simulink model "VCMGCM1962020b_v2"  (R2020b)
settings: Solver=FixedStepDiscrete  StartTime=0.0  StopTime=10.0  FixedStep=0.005  RelTol=1e-3  EnableMultiTasking=on
PreLoadFcn:
  | try, model_open; catch, disp('Error occurred while executing model pre-load callback: model_open.m'); disp('Please assure that the MATLAB working directory is set to the model directory before opening.'); end
InitFcn:
  | try, model_open; catch, end
undefined symbols (not defined in the file): Bridge, GCM, H, raptor_get_param_eval, raptor_get_safe_string, raptor_xcp_function
libraries: Blocks_lib x1165, Raptor_lib x665, simulink x62, VCM_lib x5
(part 9 of 23)

== system VCMGCM1962020b_v2/Fgnd/Control/PDU/Main  Contactor Cmd/HV Detect ==
  Data : Inport
  Abs : Abs
  Add : Sum  Inputs=+-  InputSameDT=on  OutDataTypeStr=Inherit: Same as first input
  Bus Selector : BusSelector  OutputSignals=VirtualSensors.PDU.HVBusVolt [V]
  Bus Selector1 : BusSelector  OutputSignals=VirtualSensors.Batt.BattVolt [V]
  Header : Blocks_lib/Header  width=Portrait  addtext=''
  Logical Operator : Logic  AllPortsSameDT=off  OutDataTypeStr=boolean
  Relational Operator : RelationalOperator  OutDataTypeStr=boolean  RndMeth=Nearest
  Relational Operator1 : RelationalOperator  Operator=<=  OutDataTypeStr=boolean  RndMeth=Nearest
  raptor_adjustment : Raptor_lib/Data Storage/raptor_adjustment  paramName=[nam 'PreChgHVDetectThr']  nameSource=Parameter  initValue=0  dataType=double  storage=Calibration  calDispType=Number  calEnum={'Disabled', 'Enabled'}  calGain=1  calOffset=0  calMax=inf  calMin=-inf  calFormat=''  calUnit='V'  calHelp='Pre-charge high voltage detected threshold (post contactors)'  calAccess=1  calFunction=group  calDispHeaders=off  calColHeaders={'Col1' 'Col2' 'Col3'}  calRowHeaders={'Row1' 'Row2' 'Row3'}
      settings: SourceProductName=Raptor
  raptor_adjustment1 : Raptor_lib/Data Storage/raptor_adjustment  paramName=[nam 'PreChgHVDetectDeltaThr']  nameSource=Parameter  initValue=0  dataType=double  storage=Calibration  calDispType=Number  calEnum={'Disabled', 'Enabled'}  calGain=1  calOffset=0  calMax=inf  calMin=-inf  calFormat=''  calUnit='V'  calHelp='Pre-charge high voltage detected threshold (delta between pre and post contactors)'  calAccess=1  calFunction=group  calDispHeaders=off  calColHeaders={'Col1' 'Col2' 'Col3'}  calRowHeaders={'Row1' 'Row2' 'Row3'}
      settings: SourceProductName=Raptor
  raptor_measurement : Raptor_lib/Data Storage/raptor_measurement  paramName=[nam 'HVDetect']  nameSource=Parameter  calDispType=Number  calEnum={'Disabled', 'Enabled'}  calGain=1  calOffset=0  calMax=inf  calMin=-inf  calFormat=''  calUnit='Bool'  calHelp='high voltage detected (post contactors)'  calAccess=1  calFunction=group  calVisible=on
      settings: SourceProductName=Raptor
  Full : Outport  VectorParamsAs1DForOutWhenUnconnected=off
  wires:
  raptor_adjustment1/1 -> Relational Operator1/2
  Relational Operator1/1 -> Logical Operator/2
  Relational Operator/1 -> Logical Operator/1
  Add/1 -> Abs/1
  raptor_adjustment/1 -> Relational Operator/2
  Bus Selector1/1 -> Add/2  "<BattVolt [V]>"
  Abs/1 -> Relational Operator1/1
  Logical Operator/1 -> Full/1, raptor_measurement/1
  Data/1 -> Bus Selector1/1, Bus Selector/1
  Bus Selector/1 -> Relational Operator/1, Add/1  "<HVBusVolt [V]>"

== system VCMGCM1962020b_v2/Fgnd/Control/PDU/Main  Contactor Cmd/PreCharge Sequence/EvalDiag ==
  status : Inport
  f : TriggerPort  TriggerType=function-call  VariantControl=(inherit)
      settings: CopyFcn=Stateflow.SLINSF.SimulinkMan.removeBlockPreDeleteFcn  PreDeleteFcn=Stateflow.SLINSF.SimulinkMan.unsafePredeleteFcn
  Header : Blocks_lib/Header  width=Portrait  addtext=''
  raptor_fault_def : Raptor_lib/Faults/raptor_fault_def  faultName=[nam 'PreChgFault']  persist=off  sticky=off  emisRelated=off  singleTrip=off  clearMethod=Standard  xLimit=1  yLimit=1  calEnable=on  addDisable=off  calAccess=1  calFunction=['Diagnostics | Fault Defs | ' raptor_get_param_eval(gcb, 'faultName')]
      settings: SourceProductName=Raptor
  wires:
  status/1 -> raptor_fault_def/1

== system VCMGCM1962020b_v2/Fgnd/Control/PDU/PDU Contactor Commands/CntrStatus ==
  Data : Inport
  AND : Logic  Inputs=4  AllPortsSameDT=off  OutDataTypeStr=boolean
  AND1 : Logic  Inputs=4  AllPortsSameDT=off  OutDataTypeStr=boolean
  Bus Selector : BusSelector  OutputSignals=Sensors.Sensors.Other.DrvInvtrCntrClosed.DrvInvtrCntrClosed [Bool],Sensors.Sensors.Other.DCDCCntrClosed.DCDCCntrClosedVld [Bool],Sensors.Sensors.Other.DCDCCntrClosed.DCDCCntrClosed [Bool],Sensors.Sensors.Other.ChrgrCntrClosed.ChrgrCntrClosedVld [Bool]
  Bus Selector1 : BusSelector  OutputSignals=Sensors.Sensors.Other.ChrgrCntrClosed.ChrgrCntrClosedVld [Bool],Sensors.Sensors.Other.ChrgrCntrClosed.ChrgrCntrClosed [Bool]
  Header : Blocks_lib/Header  width=Portrait  addtext=''
  Meas&Ovrd1 : Blocks_lib/Meas&Ovrd  nam='RunCntrClosed'  name_source=Parameter  view_as=Number  enum_struct={}  gain=1  min=-inf  max=inf  precision=''  units='Bool'  help='Run Contactor state'  group='Control | PDU'
  Meas&Ovrd10 : Blocks_lib/Meas&Ovrd  nam='ChrgCntrClosed'  name_source=Parameter  view_as=Number  enum_struct={}  gain=1  min=-inf  max=inf  precision=''  units='Bool'  help='Charge Contactor state'  group='Control | PDU'
  RunClosed : Outport  VectorParamsAs1DForOutWhenUnconnected=off
  ChrgClosed : Outport  Port=2  VectorParamsAs1DForOutWhenUnconnected=off
  wires:
  Data/1 -> Bus Selector1/1, Bus Selector/1
  AND1/1 -> Meas&Ovrd10/1
  AND/1 -> Meas&Ovrd1/1
  Bus Selector/1 -> AND/1  "<DrvInvtrCntrClosed [Bool]>"
  Bus Selector/2 -> AND/2  "<DCDCCntrClosedVld [Bool]>"
  Bus Selector/3 -> AND1/1, AND/3  "<DCDCCntrClosed [Bool]>"
  Bus Selector/4 -> AND1/2, AND/4  "<ChrgrCntrClosedVld [Bool]>"
  Bus Selector1/1 -> AND1/3  "<ChrgrCntrClosedVld [Bool]>"
  Bus Selector1/2 -> AND1/4  "<ChrgrCntrClosed [Bool]>"
  Meas&Ovrd10/1 -> ChrgClosed/1
  Meas&Ovrd1/1 -> RunClosed/1

== system VCMGCM1962020b_v2/Fgnd/Control/PDU/PDU Contactor Commands/Drive Inverter Contactor ==
  Data : Inport
  Abs : Abs
  Bus Selector : BusSelector  OutputSignals=Control.Mode.StartStop.RunCntr [Bool]
  Bus Selector1 : BusSelector  OutputSignals=VirtualSensors.DrvInvtr.DrvMtrSpd [rpm]
  Header : Blocks_lib/Header  width=Portrait  addtext=''
  Logical Operator : Logic  Operator=OR  AllPortsSameDT=off  OutDataTypeStr=boolean
  Logical Operator1 : Logic  Operator=NOT  Inputs=1  AllPortsSameDT=off  OutDataTypeStr=boolean
  Logical Operator2 : Logic  OutDataTypeStr=boolean
  Meas&Ovrd10 : Blocks_lib/Meas&Ovrd  nam='DrvCntrCmd'  name_source=Parameter  view_as=Number  enum_struct={}  gain=1  min=-inf  max=inf  precision=''  units='Bool'  help='Drive Contactor state'  group='Control | PDU'
  Relational Operator : RelationalOperator  Operator=>  OutDataTypeStr=boolean  RndMeth=Simplest
  Set : Blocks_lib/Set  SystemSampleTime=-1  VariantActivationTime=update diagram  Latency=0  AutoFrameSizeCalculation=off
  raptor_adjustment : Raptor_lib/Data Storage/raptor_adjustment  paramName='DrvInvtrCntrDsblMtrSpdThr'  nameSource=Parameter  initValue=0  dataType=double  storage=Calibration  calDispType=Number  calEnum={'False', 'True'}  calGain=1.0  calOffset=0.0  calMax=inf  calMin=-inf  calFormat=''  calUnit='rpm'  calHelp='Drive inverter contactor disable threshold (on motor speed, during HV discharge)'  calAccess=1  calFunction='Control | PDU'  calDispHeaders=off  calColHeaders={'Col1' 'Col2' 'Col3'}  calRowHeaders={'Row1' 'Row2' 'Row3'}
      settings: SourceProductName=Raptor
  raptor_fault_status : Raptor_lib/Faults/raptor_fault_status  faultSource=Parameter  faultName='EStop1'  notOccurred=off  suspected=off  active=off  occurred=off  failedThisDC=on  testCmpltThisDC=off  failing=off  pending=off  confirmed=off  mil=off  permanent=off  ready=off  prevConfirmed=off  failedSinceClear=off  failedLastDC=off  prevMil=off
      settings: SourceProductName=Raptor
  Bool : Outport  VectorParamsAs1DForOutWhenUnconnected=off
  wires:
  raptor_adjustment/1 -> Relational Operator/2
  Bus Selector1/1 -> Abs/1  "<DrvMtrSpd [rpm]>"
  Data/1 -> Bus Selector1/1, Bus Selector/1
  Abs/1 -> Relational Operator/1
  Bus Selector/1 -> Logical Operator2/1  "<RunCntr [Bool]>"
  Meas&Ovrd10/1 -> Bool/1
  Logical Operator2/1 -> Meas&Ovrd10/1
  Relational Operator/1 -> Logical Operator/1
  raptor_fault_status/1 -> Logical Operator/2
  Logical Operator/1 -> Set/1
  Set/1 -> Logical Operator1/1
  Logical Operator1/1 -> Logical Operator2/2

== system VCMGCM1962020b_v2/Fgnd/Control/PDU/PDU Contactor Commands/Enable ==
  Data : Inport
  Bus Selector : BusSelector  OutputSignals=Control.Mode.StartStop.RunCntr [Bool],Control.Mode.StartStop.ChgCntr [Bool]
  Header : Blocks_lib/Header  width=Portrait  addtext=''
  Logical Operator : Logic  Operator=NOT  Inputs=1  AllPortsSameDT=off  OutDataTypeStr=boolean
  Logical Operator1 : Logic  AllPortsSameDT=off  OutDataTypeStr=boolean
  Logical Operator2 : Logic  AllPortsSameDT=off  OutDataTypeStr=boolean
  raptor_fault_status : Raptor_lib/Faults/raptor_fault_status  faultSource=Parameter  faultName='EStop1'  notOccurred=off  suspected=off  active=off  occurred=off  failedThisDC=on  testCmpltThisDC=off  failing=off  pending=off  confirmed=off  mil=off  permanent=off  ready=off  prevConfirmed=off  failedSinceClear=off  failedLastDC=off  prevMil=off
      settings: SourceProductName=Raptor
  RunEnbl : Outport  VectorParamsAs1DForOutWhenUnconnected=off
  ChrgEnbl : Outport  Port=2  VectorParamsAs1DForOutWhenUnconnected=off
  wires:
  Logical Operator1/1 -> RunEnbl/1
  Data/1 -> Bus Selector/1
  Logical Operator/1 -> Logical Operator2/1, Logical Operator1/1
  raptor_fault_status/1 -> Logical Operator/1
  Bus Selector/1 -> Logical Operator1/2  "<RunCntr [Bool]>"
  Bus Selector/2 -> Logical Operator2/2  "<ChgCntr [Bool]>"
  Logical Operator2/1 -> ChrgEnbl/1

== system VCMGCM1962020b_v2/Fgnd/Control/PDU/PDU Contactor Commands/HV Detect ==
  Data : Inport
  Abs : Abs
  Add : Sum  Inputs=+-  InputSameDT=on  OutDataTypeStr=Inherit: Same as first input
  Bus Selector : BusSelector  OutputSignals=VirtualSensors.PDU.HVBusVolt [V]
  Bus Selector1 : BusSelector  OutputSignals=VirtualSensors.Batt.BattVolt [V]
  Header : Blocks_lib/Header  width=Portrait  addtext=''
  Logical Operator : Logic  AllPortsSameDT=off  OutDataTypeStr=boolean
  Relational Operator : RelationalOperator  OutDataTypeStr=boolean  RndMeth=Nearest
  Relational Operator1 : RelationalOperator  Operator=<=  OutDataTypeStr=boolean  RndMeth=Nearest
  raptor_adjustment : Raptor_lib/Data Storage/raptor_adjustment  paramName=['PreChgHVDetectThr']  nameSource=Parameter  initValue=0  dataType=double  storage=Calibration  calDispType=Number  calEnum={'Disabled', 'Enabled'}  calGain=1  calOffset=0  calMax=inf  calMin=-inf  calFormat=''  calUnit='V'  calHelp='Pre-charge high voltage detected threshold (post contactors)'  calAccess=1  calFunction=group  calDispHeaders=off  calColHeaders={'Col1' 'Col2' 'Col3'}  calRowHeaders={'Row1' 'Row2' 'Row3'}
      settings: SourceProductName=Raptor
  raptor_adjustment1 : Raptor_lib/Data Storage/raptor_adjustment  paramName=['PreChgHVDetectDeltaThr']  nameSource=Parameter  initValue=0  dataType=double  storage=Calibration  calDispType=Number  calEnum={'Disabled', 'Enabled'}  calGain=1  calOffset=0  calMax=inf  calMin=-inf  calFormat=''  calUnit='V'  calHelp='Pre-charge high voltage detected threshold (delta between pre and post contactors)'  calAccess=1  calFunction=group  calDispHeaders=off  calColHeaders={'Col1' 'Col2' 'Col3'}  calRowHeaders={'Row1' 'Row2' 'Row3'}
      settings: SourceProductName=Raptor
  raptor_measurement : Raptor_lib/Data Storage/raptor_measurement  paramName=['HVDetect']  nameSource=Parameter  calDispType=Number  calEnum={'Disabled', 'Enabled'}  calGain=1  calOffset=0  calMax=inf  calMin=-inf  calFormat=''  calUnit='Bool'  calHelp='high voltage detected (post contactors)'  calAccess=1  calFunction=group  calVisible=on
      settings: SourceProductName=Raptor
  Full : Outport  VectorParamsAs1DForOutWhenUnconnected=off
  wires:
  raptor_adjustment1/1 -> Relational Operator1/2
  Relational Operator1/1 -> Logical Operator/2
  Relational Operator/1 -> Logical Operator/1
  Add/1 -> Abs/1
  raptor_adjustment/1 -> Relational Operator/2
  Bus Selector1/1 -> Add/2  "<BattVolt [V]>"
  Abs/1 -> Relational Operator1/1
  Logical Operator/1 -> Full/1, raptor_measurement/1
  Data/1 -> Bus Selector1/1, Bus Selector/1
  Bus Selector/1 -> Relational Operator/1, Add/1  "<HVBusVolt [V]>"

== system VCMGCM1962020b_v2/Fgnd/Diagnostics/Diagnostics/A//C Compressor Fault/EvalDiag ==
  note: Note: under-voltage or internal fault are only considered a fault
      | when contactors are closed.
  Data : Inport
  Reset : EnablePort  StatesWhenEnabling=reset
  Bus Selector : BusSelector  OutputSignals=Sensors.CAN.Other.ACC.ACCSTATUS1.ACCFltStat.ACCFltStat []
  Bus Selector1 : BusSelector  OutputSignals=VirtualSensors.PDU.MainCntrClosed [Bool]
  FltTmr : Blocks_lib/FltTmr  nam='ACCFault'  tmrth_nam='ACCFaultTimeThr'  tmrth_typ=uint16  tmrth_help='Fault time threshold'  samptime=samptime  group='Diagnostics | System'
  Header : Blocks_lib/Header  width=Portrait  addtext=''
  Internal Fault : simulink/Logic and Bit Operations/Compare To Constant  relop===  const=6  OutDataTypeStr=boolean
  Logical Operator : Logic  AllPortsSameDT=off  OutDataTypeStr=boolean
  Logical Operator1 : Logic  Operator=OR  AllPortsSameDT=off  OutDataTypeStr=boolean
  Logical Operator2 : Logic  AllPortsSameDT=off  OutDataTypeStr=boolean
  Logical Operator3 : Logic  Operator=OR  AllPortsSameDT=off  OutDataTypeStr=boolean
  Logical Operator4 : Logic  Operator=NOT  AllPortsSameDT=off  OutDataTypeStr=boolean
  No Fault : simulink/Logic and Bit Operations/Compare To Zero  relop=~=  OutDataTypeStr=boolean
  Under Voltage : simulink/Logic and Bit Operations/Compare To Constant  relop===  const=1  OutDataTypeStr=boolean
  wires:
  Data/1 -> Bus Selector/1, Bus Selector1/1
  Internal Fault/1 -> Logical Operator3/2
  No Fault/1 -> Logical Operator/1
  Logical Operator/1 -> Logical Operator1/1
  Logical Operator2/1 -> Logical Operator1/2
  Under Voltage/1 -> Logical Operator3/1
  Logical Operator3/1 -> Logical Operator2/1, Logical Operator4/1
  Bus Selector1/1 -> Logical Operator2/2  "<MainCntrClosed [Bool]>"
  Logical Operator4/1 -> Logical Operator/2
  Logical Operator1/1 -> FltTmr/1
  Bus Selector/1 -> Internal Fault/1, Under Voltage/1, No Fault/1  "<ACCFltStat []>"

== system VCMGCM1962020b_v2/Fgnd/Diagnostics/Diagnostics/Battery Cell Temperature (avg) High /EvalDiag ==
  Data : Inport
  Reset : EnablePort  StatesWhenEnabling=reset
  Bus Selector : BusSelector  OutputSignals=VirtualSensors.Batt.BattCellTempAvg [degC]
  FltRngTmr : Blocks_lib/FltRngTmr  nam='BattCellTempAvgHi'  relop=>  threshnam='BattCellTempAvgHiThr'  typ=double  units='degC'  help='Range high fault threshold'  tmrth_nam='BattCellTempAvgHiTimeThr'  tmrth_typ=uint16  tmrth_help='Range high fault time threshold'  samptime=samptime  group='Diagnostics | System'
  Header : Blocks_lib/Header  width=Portrait  addtext=''
  wires:
  Data/1 -> Bus Selector/1
  Bus Selector/1 -> FltRngTmr/1  "<BattCellTempAvg [degC]>"

== system VCMGCM1962020b_v2/Fgnd/Diagnostics/Diagnostics/Battery Cell Temperature (max) High/EvalDiag ==
  Data : Inport
  Reset : EnablePort  StatesWhenEnabling=reset
  Bus Selector : BusSelector  OutputSignals=VirtualSensors.Batt.BattCellTempMx [degC]
  FltRngTmr : Blocks_lib/FltRngTmr  nam='BattCellTempMxHi'  relop=>  threshnam='BattCellTempMxHiThr'  typ=double  units='degC'  help='Range high fault threshold'  tmrth_nam='BattCellTempMxHiTimeThr'  tmrth_typ=uint16  tmrth_help='Range high fault time threshold'  samptime=samptime  group='Diagnostics | System'
  Header : Blocks_lib/Header  width=Portrait  addtext=''
  wires:
  Bus Selector/1 -> FltRngTmr/1  "<BattCellTempMx [degC]>"
  Data/1 -> Bus Selector/1

== system VCMGCM1962020b_v2/Fgnd/Diagnostics/Diagnostics/Battery Cell Voltage (max) High/EvalDiag ==
  Data : Inport
  Reset : EnablePort  StatesWhenEnabling=reset
  Bus Selector : BusSelector  OutputSignals=VirtualSensors.Batt.BattCellVoltMx [V]
  FltRngTmr : Blocks_lib/FltRngTmr  nam='BattCellVoltMxHi'  relop=>  threshnam='BattCellVoltMxHiThr'  typ=double  units='V'  help='Range high fault threshold'  tmrth_nam='BattCellVoltMxHiTimeThr'  tmrth_typ=uint16  tmrth_help='Range high fault time threshold'  samptime=samptime  group='Diagnostics | System'
  Header : Blocks_lib/Header  width=Portrait  addtext=''
  wires:
  Bus Selector/1 -> FltRngTmr/1  "<BattCellVoltMx [V]>"
  Data/1 -> Bus Selector/1

== system VCMGCM1962020b_v2/Fgnd/Diagnostics/Diagnostics/Battery Cell Voltage (min) Low/EvalDiag ==
  Data : Inport
  Reset : EnablePort  StatesWhenEnabling=reset
  Bus Selector : BusSelector  OutputSignals=VirtualSensors.Batt.BattCellVoltMn [V]
  FltRngTmr : Blocks_lib/FltRngTmr  nam='BattCellVoltMnLo'  relop=<  threshnam='BattCellVoltMnLoThr'  typ=double  units='V'  help='Range low fault threshold'  tmrth_nam='BattCellVoltMnLoTimeThr'  tmrth_typ=uint16  tmrth_help='Range low fault time threshold'  samptime=samptime  group='Diagnostics | System'
  Header : Blocks_lib/Header  width=Portrait  addtext=''
  wires:
  Data/1 -> Bus Selector/1
  Bus Selector/1 -> FltRngTmr/1  "<BattCellVoltMn [V]>"

== system VCMGCM1962020b_v2/Fgnd/Diagnostics/Diagnostics/Battery Current High/EvalDiag ==
  Data : Inport
  Reset : EnablePort  StatesWhenEnabling=reset
  Add : Sum
  Add1 : Sum
  Bus Selector1 : BusSelector  OutputSignals=VirtualSensors.Batt.BattCur [A]
  Bus Selector2 : BusSelector  OutputSignals=VirtualSensors.Batt.BattCCL [A]
  Bus Selector9 : BusSelector  OutputSignals=VirtualSensors.Batt.BattDCL [A]
  FltTmr : Blocks_lib/FltTmr  nam='BattCurHi'  tmrth_nam='BattCurHiTimeThr'  tmrth_typ=uint16  tmrth_help='Range high fault time threshold'  samptime=samptime  group='Diagnostics | System'
  Gain : Gain  Gain=-1
  Header : Blocks_lib/Header  width=Portrait  addtext=''
  Logical Operator : Logic  Operator=OR  OutDataTypeStr=boolean
  Relational Operator : RelationalOperator  Operator=>  OutDataTypeStr=boolean  RndMeth=Nearest  InputSameDT=on
  Relational Operator1 : RelationalOperator  Operator=<  OutDataTypeStr=boolean  RndMeth=Nearest  InputSameDT=on
  raptor_adjustment1 : Raptor_lib/Data Storage/raptor_adjustment  paramName='BattCurHiThrHyst'  nameSource=Parameter  initValue=0  dataType=double  storage=Calibration  calDispType=Number  calEnum={'Disabled', 'Enabled'}  calGain=1  calOffset=0  calMax=inf  calMin=-inf  calFormat=''  calUnit='A'  calHelp='Range high fault threshold hysteresis (on limits)'  calAccess=1  calFunction='Diagnostics | System'  calDispHeaders=off  calColHeaders={'Col1' 'Col2' 'Col3'}  calRowHeaders={'Row1' 'Row2' 'Row3'}
      settings: SourceProductName=Raptor
  wires:
  Add1/1 -> Gain/1
  Relational Operator/1 -> Logical Operator/1
  Relational Operator1/1 -> Logical Operator/2
  Bus Selector1/1 -> Relational Operator1/1, Relational Operator/1  "<BattCur [A]>"
  Add/1 -> Relational Operator/2
  raptor_adjustment1/1 -> Add1/2, Add/2
  Bus Selector9/1 -> Add/1  "<BattDCL [A]>"
  Bus Selector2/1 -> Add1/1  "<BattCCL [A]>"
  Logical Operator/1 -> FltTmr/1
  Gain/1 -> Relational Operator1/2
  Data/1 -> Bus Selector9/1, Bus Selector2/1, Bus Selector1/1

== system VCMGCM1962020b_v2/Fgnd/Diagnostics/Diagnostics/Battery Fault/EvalDiag ==
  Data : Inport
  Reset : EnablePort  StatesWhenEnabling=reset
  Bus Selector : BusSelector  OutputSignals=VirtualSensors.Batt.BattFault [Bool]
  FltTmr : Blocks_lib/FltTmr  nam='BattFault'  tmrth_nam='BattFaultTimeThr'  tmrth_typ=uint16  tmrth_help='Fault time threshold'  samptime=samptime  group='Diagnostics | System'
  Header : Blocks_lib/Header  width=Portrait  addtext=''
  wires:
  Data/1 -> Bus Selector/1
  Bus Selector/1 -> FltTmr/1  "<BattFault [Bool]>"

== system VCMGCM1962020b_v2/Fgnd/Diagnostics/Diagnostics/CAN Bus Passive/EvalDiag ==
  Reset : EnablePort  StatesWhenEnabling=reset
  CAN1 : Subsystem  mask{bus='CAN1'}
      mask prompts: bus "CAN Bus"
      mask init:
      | cb = gcb;
      | 
      | % --- Parameter Setting
      | set_param([cb '/raptor_can_state'], 'resource', bus);
      | set_param([cb '/raptor_can_tx_queue_info'], 'resource', bus);
      | set_param([cb '/raptor_can_tx_queue_info1'], 'resource', bus);
      mask Display: disp(bus)
  CAN2 : Subsystem  Commented=on  mask{bus='CAN2'}
      mask prompts: bus "CAN Bus"
      mask init: same as VCMGCM1962020b_v2/Fgnd/Diagnostics/Diagnostics/CAN Bus Passive/EvalDiag/CAN1
      mask Display: disp(bus)
  CAN3 : Subsystem  mask{bus='CAN3'}
      mask prompts: bus "CAN Bus"
      mask init: same as VCMGCM1962020b_v2/Fgnd/Diagnostics/Diagnostics/CAN Bus Passive/EvalDiag/CAN1
      mask Display: disp(bus)
  Header : Blocks_lib/Header  width=Portrait  addtext=''

== system VCMGCM1962020b_v2/Fgnd/Diagnostics/Diagnostics/Charger (off-board) Isolation Fault/EvalDiag ==
  Data : Inport
  Reset : EnablePort  StatesWhenEnabling=reset
  Bus Selector : BusSelector  OutputSignals=VirtualSensors.Chgr.OffBoard.OffBoardChgrIsoFault [Bool]
  FltTmr : Blocks_lib/FltTmr  nam='OffBoardChgrIsoFault'  tmrth_nam='OffBoardChgrIsoFaultTimeThr'  tmrth_typ=uint16  tmrth_help='Fault time threshold'  samptime=samptime  group='Diagnostics | System'
  Header : Blocks_lib/Header  width=Portrait  addtext=''
  wires:
  Bus Selector/1 -> FltTmr/1  "<OffBoardChgrIsoFault [Bool]>"
  Data/1 -> Bus Selector/1

== system VCMGCM1962020b_v2/Fgnd/Diagnostics/Diagnostics/Charger (on-board) Fault/EvalDiag ==
  Data : Inport
  Reset : EnablePort  StatesWhenEnabling=reset
  Bus Selector : BusSelector  OutputSignals=VirtualSensors.Chgr.OnBoard.OnBoardChgrFault [Bool]
  FltTmr : Blocks_lib/FltTmr  nam='OnBoardChgrFault'  tmrth_nam='OnBoardChgrFaultTimeThr'  tmrth_typ=uint16  tmrth_help='Fault time threshold'  samptime=samptime  group='Diagnostics | System'
  Header : Blocks_lib/Header  width=Portrait  addtext=''
  wires:
  Bus Selector/1 -> FltTmr/1  "<OnBoardChgrFault [Bool]>"
  Data/1 -> Bus Selector/1

== system VCMGCM1962020b_v2/Fgnd/Diagnostics/Diagnostics/Contactor X-Checks/EvalDiagChgrCntr ==
  Data : Inport
  Reset : EnablePort  StatesWhenEnabling=reset
  Bus Selector : BusSelector  OutputSignals=Control.PDU.PDUCntrs.ChrgrCntrCmd [Bool],VirtualSensors.PDU.ChrgrCntrClosed [Bool]
  FltTmr : Blocks_lib/FltTmr  nam='DCChgNegCntrXChk'  tmrth_nam='DCChgNegCntrXChkTimeThr'  tmrth_typ=uint16  tmrth_help='Cross-check fault time threshold'  samptime=samptime  group='Diagnostics | System'
  Header : Blocks_lib/Header  width=Portrait  addtext=''
  Logical Operator : Logic  Operator=NOT  Inputs=1  OutDataTypeStr=boolean
  Logical Operator1 : Logic  Operator=NOT  Inputs=1  OutDataTypeStr=boolean
  Logical Operator2 : Logic  OutDataTypeStr=boolean
  Logical Operator3 : Logic  OutDataTypeStr=boolean
  Logical Operator4 : Logic  Operator=OR  OutDataTypeStr=boolean
  wires:
  Data/1 -> Bus Selector/1
  Logical Operator1/1 -> Logical Operator3/1
  Logical Operator3/1 -> Logical Operator4/2
  Logical Operator2/1 -> Logical Operator4/1
  Logical Operator/1 -> Logical Operator2/2
  Bus Selector/1 -> Logical Operator2/1, Logical Operator1/1  "<ChrgrCntrCmd [Bool]>"
  Bus Selector/2 -> Logical Operator3/2, Logical Operator/1  "<ChrgrCntrClosed [Bool]>"
  Logical Operator4/1 -> FltTmr/1

== system VCMGCM1962020b_v2/Fgnd/Diagnostics/Diagnostics/Contactor X-Checks/EvalDiagDCDCCntr ==
  Data : Inport
  Reset : EnablePort  StatesWhenEnabling=reset
  Bus Selector : BusSelector  OutputSignals=VirtualSensors.PDU.DCDCCntrClosed [Bool],Control.PDU.PDUCntrs.DCDCCntrCmd [Bool]
  FltTmr : Blocks_lib/FltTmr  nam='DCChgPosCntrXChk'  tmrth_nam='DCChgPosCntrXChkTimeThr'  tmrth_typ=uint16  tmrth_help='Cross-check fault time threshold'  samptime=samptime  group='Diagnostics | System'
  Header : Blocks_lib/Header  width=Portrait  addtext=''
  Logical Operator : Logic  Operator=NOT  Inputs=1  OutDataTypeStr=boolean
  Logical Operator1 : Logic  Operator=NOT  Inputs=1  OutDataTypeStr=boolean
  Logical Operator2 : Logic  OutDataTypeStr=boolean
  Logical Operator3 : Logic  OutDataTypeStr=boolean
  Logical Operator4 : Logic  Operator=OR  OutDataTypeStr=boolean
  wires:
  Logical Operator4/1 -> FltTmr/1
  Bus Selector/2 -> Logical Operator/1, Logical Operator3/2  "<DCDCCntrCmd [Bool]>"
  Bus Selector/1 -> Logical Operator1/1, Logical Operator2/1  "<DCDCCntrClosed [Bool]>"
  Logical Operator/1 -> Logical Operator2/2
  Logical Operator2/1 -> Logical Operator4/1
  Logical Operator3/1 -> Logical Operator4/2
  Logical Operator1/1 -> Logical Operator3/1
  Data/1 -> Bus Selector/1

== system VCMGCM1962020b_v2/Fgnd/Diagnostics/Diagnostics/Contactor X-Checks/EvalDiagDrvInvtrCntr ==
  Data : Inport
  Reset : EnablePort  StatesWhenEnabling=reset
  Bus Selector : BusSelector  OutputSignals=VirtualSensors.PDU.DrvInvtrCntrClosed [Bool],Actuators.Actuators.PDU.DrvInvtrCntr.DrvInvtrCntr [Bool]
  FltTmr : Blocks_lib/FltTmr  nam='DrvInvtrCntrXChk'  tmrth_nam='DrvInvtrCntrXChkTimeThr'  tmrth_typ=uint16  tmrth_help='Cross-check fault time threshold'  samptime=samptime  group='Diagnostics | System'
  Header : Blocks_lib/Header  width=Portrait  addtext=''
  Logical Operator : Logic  Operator=NOT  Inputs=1  OutDataTypeStr=boolean
  Logical Operator1 : Logic  Operator=NOT  Inputs=1  OutDataTypeStr=boolean
  Logical Operator2 : Logic  OutDataTypeStr=boolean
  Logical Operator3 : Logic  OutDataTypeStr=boolean
  Logical Operator4 : Logic  Operator=OR  OutDataTypeStr=boolean
  wires:
  Bus Selector/2 -> Logical Operator/1, Logical Operator3/2  "<DrvInvtrCntr [Bool]>"
  Data/1 -> Bus Selector/1
  Logical Operator3/1 -> Logical Operator4/2
  Logical Operator4/1 -> FltTmr/1
  Logical Operator2/1 -> Logical Operator4/1
  Logical Operator1/1 -> Logical Operator3/1
  Bus Selector/1 -> Logical Operator1/1, Logical Operator2/1  "<DrvInvtrCntrClosed [Bool]>"
  Logical Operator/1 -> Logical Operator2/2

== system VCMGCM1962020b_v2/Fgnd/Diagnostics/Diagnostics/Contactor X-Checks/EvalDiagHVDschgCntr ==
  Data : Inport
  Reset : EnablePort  StatesWhenEnabling=reset
  Bus Selector : BusSelector  OutputSignals=VirtualSensors.PDU.HVDschgCntrClosed [Bool],Actuators.Actuators.PDU.HVDschgCntr.HVDschgCntr [Bool]
  FltTmr : Blocks_lib/FltTmr  nam='HVDschgCntrXChk'  tmrth_nam='HVDschgCntrXChkTimeThr'  tmrth_typ=uint16  tmrth_help='Cross-check fault time threshold'  samptime=samptime  group='Diagnostics | System'
  Header : Blocks_lib/Header  width=Portrait  addtext=''
  Logical Operator : Logic  Operator=NOT  Inputs=1  OutDataTypeStr=boolean
  Logical Operator1 : Logic  Operator=NOT  Inputs=1  OutDataTypeStr=boolean
  Logical Operator2 : Logic  OutDataTypeStr=boolean
  Logical Operator3 : Logic  OutDataTypeStr=boolean
  Logical Operator4 : Logic  Operator=OR  OutDataTypeStr=boolean
  wires:
  Logical Operator4/1 -> FltTmr/1
  Bus Selector/2 -> Logical Operator/1, Logical Operator3/2  "<HVDschgCntr [Bool]>"
  Bus Selector/1 -> Logical Operator1/1, Logical Operator2/1  "<HVDschgCntrClosed [Bool]>"
  Logical Operator/1 -> Logical Operator2/2
  Logical Operator2/1 -> Logical Operator4/1
  Logical Operator3/1 -> Logical Operator4/2
  Logical Operator1/1 -> Logical Operator3/1
  Data/1 -> Bus Selector/1

== system VCMGCM1962020b_v2/Fgnd/Diagnostics/Diagnostics/Contactor X-Checks/EvalDiagInvtrCntr ==
  Data : Inport
  Reset : EnablePort  StatesWhenEnabling=reset
  Bus Selector : BusSelector  OutputSignals=Control.PDU.PDUCntrs.DrvInvtrCntrCmd [Bool],VirtualSensors.PDU.HVDschgCntrClosed [Bool]
  FltTmr : Blocks_lib/FltTmr  nam='MainNegCntrXChk'  tmrth_nam='MainNegCntrXChkTimeThr'  tmrth_typ=uint16  tmrth_help='Cross-check fault time threshold'  samptime=samptime  group='Diagnostics | System'
  Header : Blocks_lib/Header  width=Portrait  addtext=''
  Logical Operator : Logic  Operator=NOT  Inputs=1  OutDataTypeStr=boolean
  Logical Operator1 : Logic  Operator=NOT  Inputs=1  OutDataTypeStr=boolean
  Logical Operator2 : Logic  OutDataTypeStr=boolean
  Logical Operator3 : Logic  OutDataTypeStr=boolean
  Logical Operator4 : Logic  Operator=OR  OutDataTypeStr=boolean
  wires:
  Data/1 -> Bus Selector/1
  Logical Operator1/1 -> Logical Operator3/1
  Logical Operator3/1 -> Logical Operator4/2
  Logical Operator2/1 -> Logical Operator4/1
  Logical Operator/1 -> Logical Operator2/2
  Bus Selector/1 -> Logical Operator2/1, Logical Operator1/1  "<DrvInvtrCntrCmd [Bool]>"
  Bus Selector/2 -> Logical Operator3/2, Logical Operator/1  "<HVDschgCntrClosed [Bool]>"
  Logical Operator4/1 -> FltTmr/1

== system VCMGCM1962020b_v2/Fgnd/Diagnostics/Diagnostics/Contactor X-Checks/EvalDiagMainCntr ==
  Data : Inport
  Reset : EnablePort  StatesWhenEnabling=reset
  Bus Selector : BusSelector  OutputSignals=VirtualSensors.PDU.MainPosCntrClosed [Bool],Control.Mode.StartStop.MainCntrReq [Bool]
  FltTmr : Blocks_lib/FltTmr  nam='MainPosCntrXChk'  tmrth_nam='MainPosCntrXChkTimeThr'  tmrth_typ=uint16  tmrth_help='Cross-check fault time threshold'  samptime=samptime  group='Diagnostics | System'
  Header : Blocks_lib/Header  width=Portrait  addtext=''
  Logical Operator : Logic  Operator=NOT  Inputs=1  OutDataTypeStr=boolean
  Logical Operator1 : Logic  Operator=NOT  Inputs=1  OutDataTypeStr=boolean
  Logical Operator2 : Logic  OutDataTypeStr=boolean
  Logical Operator3 : Logic  OutDataTypeStr=boolean
  Logical Operator4 : Logic  Operator=OR  OutDataTypeStr=boolean
  wires:
  Logical Operator4/1 -> FltTmr/1
  Bus Selector/2 -> Logical Operator/1, Logical Operator3/2  "<MainCntrReq [Bool]>"
  Bus Selector/1 -> Logical Operator1/1, Logical Operator2/1  "<MainPosCntrClosed [Bool]>"
  Logical Operator/1 -> Logical Operator2/2
  Logical Operator2/1 -> Logical Operator4/1
  Logical Operator3/1 -> Logical Operator4/2
  Logical Operator1/1 -> Logical Operator3/1
  Data/1 -> Bus Selector/1

== system VCMGCM1962020b_v2/Fgnd/Diagnostics/Diagnostics/Cooling Pump Fault/EvalDiag1 ==
  Data : Inport
  Reset : EnablePort  StatesWhenEnabling=reset
  Bus Selector : BusSelector  OutputSignals=Sensors.CAN.Other.CoolPump1.CoolPump1DM1.CoolPump1SPN [enum]
  Compare To Constant : simulink/Logic and Bit Operations/Compare To Constant  relop=~=  const=0  OutDataTypeStr=boolean
  FltTmr : Blocks_lib/FltTmr  nam='CoolPump1Fault'  tmrth_nam='CoolPump1FaultTimeThr'  tmrth_typ=uint16  tmrth_help='Fault time threshold'  samptime=samptime  group='Diagnostics | System'
  Header : Blocks_lib/Header  width=Portrait  addtext=''
  Logical Operator : Logic  Operator=OR  Inputs=1  OutDataTypeStr=boolean
  wires:
  Logical Operator/1 -> FltTmr/1
  Bus Selector/1 -> Compare To Constant/1  "<CoolPump1SPN [enum]>"
  Compare To Constant/1 -> Logical Operator/1
  Data/1 -> Bus Selector/1

== system VCMGCM1962020b_v2/Fgnd/Diagnostics/Diagnostics/Cooling Pump Fault/EvalDiag2 ==
  Data : Inport
  Reset : EnablePort  StatesWhenEnabling=reset
  Bus Selector : BusSelector  OutputSignals=Sensors.CAN.Other.CoolPump2.CoolPump2DM1.CoolPump2SPN [enum]
  Compare To Constant : simulink/Logic and Bit Operations/Compare To Constant  relop=~=  const=0  OutDataTypeStr=boolean
  FltTmr : Blocks_lib/FltTmr  nam='CoolPump2Fault'  tmrth_nam='CoolPump2FaultTimeThr'  tmrth_typ=uint16  tmrth_help='Fault time threshold'  samptime=samptime  group='Diagnostics | System'
  Header : Blocks_lib/Header  width=Portrait  addtext=''
  Logical Operator : Logic  Operator=OR  Inputs=1  OutDataTypeStr=boolean
  wires:
  Data/1 -> Bus Selector/1
  Compare To Constant/1 -> Logical Operator/1
  Bus Selector/1 -> Compare To Constant/1  "<CoolPump2SPN [enum]>"
  Logical Operator/1 -> FltTmr/1

== system VCMGCM1962020b_v2/Fgnd/Diagnostics/Diagnostics/DC//DC Converter Fault/EvalDiag ==
  Data : Inport
  Reset : EnablePort  StatesWhenEnabling=reset
  Bus Selector : BusSelector  OutputSignals=VirtualSensors.DCDC.DCDCFault [Bool]
  FltTmr : Blocks_lib/FltTmr  nam='DCDCFault'  tmrth_nam='DCDCFaultTimeThr'  tmrth_typ=uint16  tmrth_help='Fault time threshold'  samptime=samptime  group='Diagnostics | System'
  Header : Blocks_lib/Header  width=Portrait  addtext=''
  wires:
  Bus Selector/1 -> FltTmr/1  "<DCDCFault [Bool]>"
  Data/1 -> Bus Selector/1

== system VCMGCM1962020b_v2/Fgnd/Diagnostics/Diagnostics/DC//DC Converter X-Check/EvalDiag ==
  Data : Inport
  Reset : EnablePort  StatesWhenEnabling=reset
  Add : Sum  Inputs=+-
  Bus Selector : BusSelector  OutputSignals=Sensors.Sensors.Volt.DRVPVolt.DRVPVolt [V],Control.DCDC.DCDCOutptVoltSetpt [V]
  FltRngTmr : Blocks_lib/FltRngTmr  nam='DCDCXChk'  relop=<  threshnam='DCDCXChkThr'  typ=double  units='V'  help='Cross-check fault threshold'  tmrth_nam='DCDCXChkTimeThr'  tmrth_typ=uint16  tmrth_help='Cross-check fault time threshold'  samptime=samptime  group='Diagnostics | System'
  Header : Blocks_lib/Header  width=Portrait  addtext=''
  wires:
  Bus Selector/2 -> Add/2  "<DCDCOutptVoltSetpt [V]>"
  Bus Selector/1 -> Add/1  "<DRVPVolt [V]>"
  Add/1 -> FltRngTmr/1
  Data/1 -> Bus Selector/1

== system VCMGCM1962020b_v2/Fgnd/Diagnostics/Diagnostics/DRVP Voltage High//Low/EvalDiag ==
  Data : Inport
  Reset : EnablePort  StatesWhenEnabling=reset
  Bus Selector : BusSelector  OutputSignals=Sensors.Sensors.Volt.DRVPVolt.DRVPVolt [V]
  FltRngTmr : Blocks_lib/FltRngTmr  nam='DRVPVoltHi'  relop=>  threshnam='DRVPVoltHiThr'  typ=double  units='V'  help='Range high fault threshold'  tmrth_nam='DRVPVoltHiTimeThr'  tmrth_typ=uint16  tmrth_help='Range high fault time threshold'  samptime=samptime  group='Diagnostics | System'
  FltRngTmr1 : Blocks_lib/FltRngTmr  nam='DRVPVoltLo'  relop=<  threshnam='DRVPVoltLoThr'  typ=double  units='V'  help='Range low fault threshold'  tmrth_nam='DRVPVoltLoTimeThr'  tmrth_typ=uint16  tmrth_help='Range low fault time threshold'  samptime=samptime  group='Diagnostics | System'
  Header : Blocks_lib/Header  width=Portrait  addtext=''
  wires:
  Data/1 -> Bus Selector/1
  Bus Selector/1 -> FltRngTmr/1, FltRngTmr1/1  "<DRVPVolt [V]>"

== system VCMGCM1962020b_v2/Fgnd/Diagnostics/Diagnostics/Drive Inverter Fault/EvalDiag ==
  Data : Inport
  Reset : EnablePort  StatesWhenEnabling=reset
  Bus Selector : BusSelector  OutputSignals=VirtualSensors.DrvInvtr.DrvInvtrFault [Bool]
  FltTmr : Blocks_lib/FltTmr  nam='DrvInvtrFault'  tmrth_nam='DrvInvtrFaultTimeThr'  tmrth_typ=uint16  tmrth_help='Fault time threshold'  samptime=samptime  group='Diagnostics | System'
  Header : Blocks_lib/Header  width=Portrait  addtext=''
  wires:
  Data/1 -> Bus Selector/1
  Bus Selector/1 -> FltTmr/1  "<DrvInvtrFault [Bool]>"

== system VCMGCM1962020b_v2/Fgnd/Diagnostics/Diagnostics/Drive Motor Torque X-Check/EvalDiag ==
  Data : Inport
  Reset : EnablePort  StatesWhenEnabling=reset
  Add : Sum  Inputs=+-
  Bus Selector : BusSelector  OutputSignals=VirtualSensors.DrvInvtr.DrvMtrTrq [Nm],Control.DrvInvtr.MtrTrqReq.DrvInvtr.DrvMtrTrqReq [Nm]
  Compare To Zero : simulink/Logic and Bit Operations/Compare To Zero  relop=<  OutDataTypeStr=boolean
  FltRngTmr : Blocks_lib/FltRngTmr  nam='DrvMtrTrqHi'  relop=>  threshnam='DrvMtrTrqHiThr'  typ=double  units='Nm'  help='Cross-check fault threshold'  tmrth_nam='DrvMtrTrqHiTimeThr'  tmrth_typ=uint16  tmrth_help='Cross-check fault time threshold'  samptime=samptime  group='Diagnostics | System'
  FltRngTmr1 : Blocks_lib/FltRngTmr  nam='DrvMtrTrqLo'  relop=<  threshnam='DrvMtrTrqLoThr'  typ=double  units='Nm'  help='Cross-check fault threshold'  tmrth_nam='DrvMtrTrqLoTimeThr'  tmrth_typ=uint16  tmrth_help='Cross-check fault time threshold'  samptime=samptime  group='Diagnostics | System'
  Gain : Gain  Gain=-1
  Header : Blocks_lib/Header  width=Portrait  addtext=''
  Multiport Switch : MultiPortSwitch  DataPortOrder=Zero-based contiguous  Inputs=2  zeroidx=on
  wires:
  Data/1 -> Bus Selector/1
  Bus Selector/1 -> Add/1  "<DrvMtrTrq [Nm]>"
  Bus Selector/2 -> Add/2, Compare To Zero/1  "<DrvMtrTrqReq [Nm]>"
  Compare To Zero/1 -> Multiport Switch/1
  Gain/1 -> Multiport Switch/3
  Add/1 -> Multiport Switch/2, Gain/1
  Multiport Switch/1 -> FltRngTmr/1, FltRngTmr1/1

== system VCMGCM1962020b_v2/Fgnd/Diagnostics/Diagnostics/E-Stop/EvalDiag1 ==
  Data : Inport
  Reset : EnablePort  StatesWhenEnabling=reset
  Bus Selector : BusSelector  OutputSignals=Sensors.Sensors.Driver.EStop1.EStop1 [Bool]
  Header : Blocks_lib/Header  width=Portrait  addtext=''
  raptor_fault_def : Raptor_lib/Faults/raptor_fault_def  faultName='EStop1'  persist=off  sticky=off  emisRelated=off  singleTrip=off  clearMethod=Standard  xLimit=1  yLimit=1  calEnable=on  addDisable=off  calAccess=1  calFunction=['Diagnostics | Fault Defs | ' raptor_get_param_eval(gcb, 'faultName')]
      settings: SourceProductName=Raptor
  wires:
  Data/1 -> Bus Selector/1
  Bus Selector/1 -> raptor_fault_def/1  "<EStop1 [Bool]>"

== system VCMGCM1962020b_v2/Fgnd/Diagnostics/Diagnostics/E-Stop/EvalDiag2 ==
  Data : Inport
  Reset : EnablePort  StatesWhenEnabling=reset
  Bus Selector : BusSelector  OutputSignals=Sensors.Sensors.Driver.EStop2.EStop2 [Bool]
  Header : Blocks_lib/Header  width=Portrait  addtext=''
  raptor_fault_def : Raptor_lib/Faults/raptor_fault_def  faultName='EStop2'  persist=off  sticky=off  emisRelated=off  singleTrip=off  clearMethod=Standard  xLimit=1  yLimit=1  calEnable=on  addDisable=off  calAccess=1  calFunction=['Diagnostics | Fault Defs | ' raptor_get_param_eval(gcb, 'faultName')]
      settings: SourceProductName=Raptor
  wires:
  Bus Selector/1 -> raptor_fault_def/1  "<EStop2 [Bool]>"
  Data/1 -> Bus Selector/1

== system VCMGCM1962020b_v2/Fgnd/Diagnostics/Diagnostics/HV Bus Isolation Low/EvalDiag ==
  Data : Inport
  Reset : EnablePort  StatesWhenEnabling=reset
  Bus Selector : BusSelector  OutputSignals=VirtualSensors.PDU.ISOFailed [Bool]
  Data Type Conversion : DataTypeConversion  OutDataTypeStr=uint8
  FltRngTmr : Blocks_lib/FltRngTmr  nam='HVBusISO'  relop===  threshnam='HVBusISOFaltState'  typ=uint8  units='V'  help='State that equals fault condition'  tmrth_nam='HVBusISOFaltStateTimeThr'  tmrth_typ=uint16  tmrth_help=' time threshold'  samptime=samptime  group='Diagnostics | System'
  Header : Blocks_lib/Header  width=Portrait  addtext=''
  wires:
  Data/1 -> Bus Selector/1
  Data Type Conversion/1 -> FltRngTmr/1
  Bus Selector/1 -> Data Type Conversion/1  "<ISOFailed [Bool]>"

== system VCMGCM1962020b_v2/Fgnd/Diagnostics/Diagnostics/HV Bus Voltage High/EvalDiag ==
  Data : Inport
  Reset : EnablePort  StatesWhenEnabling=reset
  Bus Selector : BusSelector  OutputSignals=VirtualSensors.PDU.HVBusVolt [V]
  FltRngTmr : Blocks_lib/FltRngTmr  nam='HVBusVoltHi'  relop=>  threshnam='HVBusVoltHiThr'  typ=double  units='V'  help='Range high fault threshold'  tmrth_nam='HVBusVoltHiTimeThr'  tmrth_typ=uint16  tmrth_help='Range high fault time threshold'  samptime=samptime  group='Diagnostics | System'
  Header : Blocks_lib/Header  width=Portrait  addtext=''
  wires:
  Bus Selector/1 -> FltRngTmr/1  "<HVBusVolt [V]>"
  Data/1 -> Bus Selector/1

== system VCMGCM1962020b_v2/Fgnd/Diagnostics/Diagnostics/HVIL X-Check/EvalDiag ==
  Data : Inport
  Reset : EnablePort  StatesWhenEnabling=reset
  Abs : Abs
  Add : Sum  Inputs=+-  InputSameDT=on  OutDataTypeStr=Inherit: Same as first input
  Bus Selector4 : BusSelector  OutputSignals=Sensors.Sensors.Other.HVILInFrq [Hz],Control.Other.Other.HVILOutFrq [Hz]
  HVIL X-Check : Stateflow chart  TreatAsAtomicUnit=on
  Header : Blocks_lib/Header  width=Portrait  addtext=''
  Relational Operator : RelationalOperator  Operator=>  OutDataTypeStr=boolean  RndMeth=Nearest  InputSameDT=on
  raptor_adjustment : Raptor_lib/Data Storage/raptor_adjustment  paramName='HVILXChkThr'  nameSource=Parameter  initValue=0  dataType=double  storage=Calibration  calDispType=Number  calEnum={'Disabled', 'Enabled'}  calGain=1  calOffset=0  calMax=inf  calMin=-inf  calFormat=''  calUnit='Hz'  calHelp='Cross-check fault threshold'  calAccess=1  calFunction='Diagnostics | System'  calDispHeaders=off  calColHeaders={'Col1' 'Col2' 'Col3'}  calRowHeaders={'Row1' 'Row2' 'Row3'}
      settings: SourceProductName=Raptor
  raptor_adjustment1 : Raptor_lib/Data Storage/raptor_adjustment  paramName='HVILXChkTimeThr'  nameSource=Parameter  initValue=0  dataType=uint16  storage=Calibration  calDispType=Number  calEnum={'Disabled', 'Enabled'}  calGain=samptime  calOffset=0  calMax=inf  calMin=-inf  calFormat='0.3'  calUnit='sec'  calHelp='Cross-check fault time threshold'  calAccess=1  calFunction='Diagnostics | System'  calDispHeaders=off  calColHeaders={'Col1' 'Col2' 'Col3'}  calRowHeaders={'Row1' 'Row2' 'Row3'}
      settings: SourceProductName=Raptor
  wires:
  Abs/1 -> Relational Operator/1
  Add/1 -> Abs/1
  Bus Selector4/1 -> Add/1  "<HVILInFrq [Hz]>"
  Bus Selector4/2 -> Add/2  "<HVILOutFrq [Hz]>"
  raptor_adjustment1/1 -> HVIL X-Check/2(FaultTimeThr)
  raptor_adjustment/1 -> Relational Operator/2
  Relational Operator/1 -> HVIL X-Check/1(Sus)
  Data/1 -> Bus Selector4/1

== system VCMGCM1962020b_v2/Fgnd/Diagnostics/Diagnostics/Heater Fault/EvalDiag ==
  note: Note: under-voltage is only considered a fault
      | when contactors are closed.
  Data : Inport
  Reset : EnablePort  StatesWhenEnabling=reset
  Bitwise Operator : simulink/Logic and Bit Operations/Bitwise Operator  logicop=AND  UseBitMask=on  BitMask=bin2dec('011111111111')  BitMaskRealWorld=Stored Integer
  Bus Selector : BusSelector  OutputSignals=Sensors.CAN.Other.Heater.HTR_OUT_1.HTR_STAT.HTR_STAT []
  Bus Selector1 : BusSelector  OutputSignals=VirtualSensors.PDU.MainCntrClosed [Bool]
  Compare To Zero : simulink/Logic and Bit Operations/Compare To Zero  relop=~=  OutDataTypeStr=boolean
  FltTmr : Blocks_lib/FltTmr  nam='HeaterFault'  tmrth_nam='HeaterFaultTimeThr'  tmrth_typ=uint16  tmrth_help='Fault time threshold'  samptime=samptime  group='Diagnostics | System'
  Header : Blocks_lib/Header  width=Portrait  addtext=''
  Logical Operator : Logic  AllPortsSameDT=off  OutDataTypeStr=boolean
  Logical Operator1 : Logic  Operator=OR  AllPortsSameDT=off  OutDataTypeStr=boolean
  Logical Operator2 : Logic  AllPortsSameDT=off  OutDataTypeStr=boolean
  Logical Operator4 : Logic  Operator=NOT  AllPortsSameDT=off  OutDataTypeStr=boolean
  Over Voltage or Under Voltage of HV System : simulink/Logic and Bit Operations/Bitwise Operator  logicop=AND  UseBitMask=on  BitMask=bin2dec('1000')  BitMaskRealWorld=Stored Integer
  wires:
  Bitwise Operator/1 -> Compare To Zero/1
  Bus Selector/1 -> Over Voltage or Under Voltage of HV System/1, Bitwise Operator/1  "<HTR_STAT []>"
  Logical Operator2/1 -> Logical Operator1/2
  Logical Operator4/1 -> Logical Operator/2
  Logical Operator/1 -> Logical Operator1/1
  Compare To Zero/1 -> Logical Operator/1
  Bus Selector1/1 -> Logical Operator2/2  "<MainCntrClosed [Bool]>"
  Over Voltage or Under Voltage of HV System/1 -> Logical Operator2/1, Logical Operator4/1
  Data/1 -> Bus Selector/1, Bus Selector1/1
  Logical Operator1/1 -> FltTmr/1

== system VCMGCM1962020b_v2/Fgnd/Diagnostics/Diagnostics/Inertia Switch/EvalDiag ==
  Data : Inport
  Reset : EnablePort  StatesWhenEnabling=reset
  Bus Selector : BusSelector  OutputSignals=Sensors.Sensors.Other.InertiaSw.InertiaSw [Bool]
  Header : Blocks_lib/Header  width=Portrait  addtext=''
  raptor_fault_def : Raptor_lib/Faults/raptor_fault_def  faultName='InertiaSw'  persist=off  sticky=off  emisRelated=off  singleTrip=off  clearMethod=Standard  xLimit=1  yLimit=1  calEnable=on  addDisable=off  calAccess=1  calFunction=['Diagnostics | Fault Defs | ' raptor_get_param_eval(gcb, 'faultName')]
      settings: SourceProductName=Raptor
  wires:
  Bus Selector/1 -> raptor_fault_def/1  "<InertiaSw [Bool]>"
  Data/1 -> Bus Selector/1

== system VCMGCM1962020b_v2/Fgnd/Diagnostics/Diagnostics/MPDM Fuse & Relay Faults/MPDM Fuse Faults ==
  Data : Inport
  Reset : EnablePort  StatesWhenEnabling=reset
  Bus Selector : BusSelector  OutputSignals=Sensors.CAN.Other.MPDM.MPDMFuseStatus.MPDMFuse1Status.MPDMFuse1Status [],Sensors.CAN.Other.MPDM.MPDMFuseStatus.MPDMFuse2Status.MPDMFuse2Status [],Sensors.CAN.Other.MPDM.MPDMFuseStatus.MPDMFuse4Status.MPDMFuse4Status [],Sensors.CAN.Other.MPDM.MPDMFuseStatus.MPDMFuse7Status.MPDMFuse7Status [],Sensors.CAN.Other.MPDM.MPDMFuseStatus.MPDMFuse8Status.MPDMFuse8Status []
  Header : Blocks_lib/Header  width=Portrait  addtext=''
  MPDMFuseFlt : Blocks_lib/MPDMFuseFlt  nam='SysWake'
  MPDMFuseFlt1 : Blocks_lib/MPDMFuseFlt  nam='HeaterPump'
  MPDMFuseFlt2 : Blocks_lib/MPDMFuseFlt  nam='PrkPawl'
  MPDMFuseFlt3 : Blocks_lib/MPDMFuseFlt  nam='BrkVacuumPump'
  MPDMFuseFlt4 : Blocks_lib/MPDMFuseFlt  nam='CoolFan'
  wires:
  Bus Selector/5 -> MPDMFuseFlt4/1  "<MPDMFuse8Status []>"
  Bus Selector/4 -> MPDMFuseFlt3/1  "<MPDMFuse7Status []>"
  Bus Selector/3 -> MPDMFuseFlt2/1  "<MPDMFuse4Status []>"
  Data/1 -> Bus Selector/1
  Bus Selector/1 -> MPDMFuseFlt/1  "<MPDMFuse1Status []>"
  Bus Selector/2 -> MPDMFuseFlt1/1  "<MPDMFuse2Status []>"

== system VCMGCM1962020b_v2/Fgnd/Diagnostics/Diagnostics/MPDM Fuse & Relay Faults/MPDM Relay Faults ==
  Data : Inport
  Reset : EnablePort  StatesWhenEnabling=reset
  Bus Selector : BusSelector  OutputSignals=Sensors.CAN.Other.MPDM.MPDMRelayStatus.MPDMRelay1Status.MPDMRelay1Status [],Sensors.CAN.Other.MPDM.MPDMRelayStatus.MPDMRelay2Status.MPDMRelay2Status [],Sensors.CAN.Other.MPDM.MPDMRelayStatus.MPDMRelay3Status.MPDMRelay3Status [],Sensors.CAN.Other.MPDM.MPDMRelayStatus.MPDMRelay4Status.MPDMRelay4Status [],Sensors.CAN.Other.MPDM.MPDMRelayStatus.MPDMRelay5Status.MPDMRelay5Status []
  Header : Blocks_lib/Header  width=Portrait  addtext=''
  MPDMRelayFlt : Blocks_lib/MPDMRelayFlt  nam='SysWake'
  MPDMRelayFlt1 : Blocks_lib/MPDMRelayFlt  nam='PrkPawl'
  MPDMRelayFlt2 : Blocks_lib/MPDMRelayFlt  nam='BrkVacuumPump'
  MPDMRelayFlt3 : Blocks_lib/MPDMRelayFlt  nam='HeaterPump'
  MPDMRelayFlt4 : Blocks_lib/MPDMRelayFlt  nam='CoolFan'
  wires:
  Data/1 -> Bus Selector/1
  Bus Selector/1 -> MPDMRelayFlt/1  "<MPDMRelay1Status []>"
  Bus Selector/2 -> MPDMRelayFlt1/1  "<MPDMRelay2Status []>"
  Bus Selector/3 -> MPDMRelayFlt2/1  "<MPDMRelay3Status []>"
  Bus Selector/4 -> MPDMRelayFlt3/1  "<MPDMRelay4Status []>"
  Bus Selector/5 -> MPDMRelayFlt4/1  "<MPDMRelay5Status []>"

== system VCMGCM1962020b_v2/Fgnd/Diagnostics/Diagnostics/MPRD Open//Short/EvalDiag ==
  Reset : EnablePort  StatesWhenEnabling=reset
  FltTmr : Blocks_lib/FltTmr  nam='MPRDOpnShrt'  tmrth_nam='MPRDOpnShrtTimeThr'  tmrth_typ=uint16  tmrth_help='Output open/shorted fault time threshold'  samptime=samptime  group='Diagnostics | Actuators'
  Header : Blocks_lib/Header  width=Portrait  addtext=''
  Terminator : Terminator
  raptor_output_status : Raptor_lib/Input & Output/raptor_output_status  resourceValues=OUTPUT13|OUTPUT14|OUTPUT15|OUTPUT16|OUTPUT17|OUTPUT18|OUTPUT19|OUTPUT20|OUTPUT56|OUTPUT57|OUTPUT58|OUTPUT59|OUTPUT60|OUTPUT61|OUTPUT62|OUTPUT63|OUTPUT1|OUTPUT2|OUTPUT3|OUTPUT4|OUTPUT5|OUTPUT6|OUTPUT7|OUTPUT8|OUTPUT9|OUTPUT10|OUTPUT11|OUTPUT12|OUTPUT21|OUTPUT22|OUTPUT23|OUTPUT24|OUTPUT25|OUTPUT26|OUTPUT27|OUTPUT28|OUTPUT29|OUTPUT30|OUTPUT31|OUTPUT32|OUTPUT33|OUTPUT34|OUTPUT35|OUTPUT36|OUTPUT37|OUTPUT38|OUTPUT39|OUTPUT40|OUTPUT41|OUTPUT42|OUTPUT43|OUTPUT44|OUTPUT45|OUTPUT46|OUTPUT47|OUTPUT48|OUTPUT49|OUTPUT50_51|OUTPUT52_53|OUTPUT54_55|MPRD|VSENS_SUPPLY1|VSENS_SUPPLY2|VSENS_SUPPLY3|(None)  resource=MPRD
      settings: SourceProductName=Raptor
  wires:
  raptor_output_status/2 -> Terminator/1
  raptor_output_status/1 -> FltTmr/1

== system VCMGCM1962020b_v2/Fgnd/Diagnostics/Diagnostics/Power Steering Pump Inverter Fault/EvalDiag ==
  Data : Inport
  Reset : EnablePort  StatesWhenEnabling=reset
  Bus Selector : BusSelector  OutputSignals=Sensors.CAN.Other.PSPInvtr.PSPInvtrHS2_Status_Feedback.PSPInvtrInverterStatus.PSPInvtrInverterStatus [enum]
  Enabled : simulink/Logic and Bit Operations/Compare To Constant  relop=~=  const=8  OutDataTypeStr=boolean
  FltTmr : Blocks_lib/FltTmr  nam='PSPInvtrFault'  tmrth_nam='PSPInvtrFaultTimeThr'  tmrth_typ=uint16  tmrth_help='Fault time threshold'  samptime=samptime  group='Diagnostics | System'
  Header : Blocks_lib/Header  width=Portrait  addtext=''
  Logical Operator : Logic  AllPortsSameDT=off  OutDataTypeStr=boolean
  Shutdown : simulink/Logic and Bit Operations/Compare To Constant  relop=~=  const=2  OutDataTypeStr=boolean
  wires:
  Logical Operator/1 -> FltTmr/1
  Enabled/1 -> Logical Operator/2
  Shutdown/1 -> Logical Operator/1
  Bus Selector/1 -> Shutdown/1, Enabled/1  "<PSPInvtrInverterStatus [enum]>"
  Data/1 -> Bus Selector/1

== system VCMGCM1962020b_v2/Fgnd/Diagnostics/Diagnostics/XDRP Voltage High//Low/EvalDiag ==
  Data : Inport
  Reset : EnablePort  StatesWhenEnabling=reset
  Bus Selector : BusSelector  OutputSignals=Sensors.Sensors.Volt.XDRPVolt.XDRPVolt [V]
  FltRngTmr : Blocks_lib/FltRngTmr  nam='XDRPVoltHi'  relop=>  threshnam='XDRPVoltHiThr'  typ=double  units='V'  help='Range high fault threshold'  tmrth_nam='XDRPVoltHiTimeThr'  tmrth_typ=uint16  tmrth_help='Range high fault time threshold'  samptime=samptime  group='Diagnostics | System'
  FltRngTmr1 : Blocks_lib/FltRngTmr  nam='XDRPVoltLo'  relop=<  threshnam='XDRPVoltLoThr'  typ=double  units='V'  help='Range low fault threshold'  tmrth_nam='XDRPVoltLoTimeThr'  tmrth_typ=uint16  tmrth_help='Range low fault time threshold'  samptime=samptime  group='Diagnostics | System'
  Header : Blocks_lib/Header  width=Portrait  addtext=''
  wires:
  Data/1 -> Bus Selector/1
  Bus Selector/1 -> FltRngTmr/1, FltRngTmr1/1  "<XDRPVolt [V]>"
